simulink model "DCDCconverter"  (R2012b)
settings: Solver=ode3  StartTime=0.0  StopTime=inf  FixedStep=Tsample_simulink  RelTol=1e-3
PostLoadFcn:
  | , if any(exist('dsrtsu_mdlpostloadfcn', 'file') == [2, 3, 6]), try dsrtsu_mdlpostloadfcn('Execute', bdroot); catch fprintf('Error in PostLoadFcn (dsrtsu_mdlpostloadfcn) for model "%s":\n %s\n', bdroot, lasterr); end, end,
InitFcn:
  | load('../sim/me547_based_PI_controller_v3_saved_state.mat');
  | load('../sim/RuleBasedControlData_LiFe_76p8V_0C.mat');
undefined symbols (not defined in the file): BatVoltageLowerThresh, BatVoltageUpperThresh, C, DiscIntNeverNeededParam, Ea, fdesignblkfcn, gcbh, Icommand_Limit, Ireg_Integ_Limit, Kp_vc, MaxBatCurrent, MaxBatVoltage, MaxTemperature, MaxUCCurrent, MaxUCVoltage, Ra, RuleBasedControlHESSPowerValues, RuleBasedControlLUTValues, RuleBasedControlUCVoltageValues, TDelay_UltracapacitorRelay, Ts, Ts2, Tsample_simulink, UCVoltageLowerThresh, UCVoltageUpperThresh, Vbat, Vrail_rated
libraries: xpclib x35, rtilib1103 x8, dspsigops x5
(part 2 of 10)

== system DCDCconverter/RTI Data/RTI Data Store ==
  RTI Data Store : Subsystem  mask(RTI_DATA_STORE){}
      mask help:
      | RTI Data Store Block. This block is used by RTI to store internal model dependent data. Deleting this block will result in data loss.
      |
      | NEVER DELETE, COPY, OR MODIFY THIS BLOCK!
      mask Help:
      | RTI Data Store Block. This block is used by RTI to store internal model dependent data. Deleting this block will result in data loss.
      | 
      | NEVER DELETE, COPY, OR MODIFY THIS BLOCK!
      mask Display: text(0.5, 0.5, ' ', 'HorizontalAlignment', 'center');

== system DCDCconverter/Test Icmd/RuleBasedControlWithLUT ==
  HESSPower : Inport
  UCVoltage : Inport  Port=2
  2-D Lookup Table : Lookup_n-D  BreakpointsForDimension1=RuleBasedControlHESSPowerValues  BreakpointsForDimension2=RuleBasedControlUCVoltageValues  BreakpointsForDimension1Min=0  BreakpointsForDimension1Max=20000  Table=RuleBasedControlLUTValues  RndMeth=Simplest  InputSameDT=on
  MATLAB Function1 : MATLAB Function  TreatAsAtomicUnit=on
  Ra : Gain  Gain=-1
  Saturation : Saturate  UpperLimit=0  LowerLimit=-Icommand_Limit
  Switch2 : Switch  Threshold=1  OutDataTypeStr=Inherit: Inherit via back propagation
  UCCurrentCommand : Outport
  wires:
  HESSPower/1 -> MATLAB Function1/2(Pout), 2-D Lookup Table/1
  2-D Lookup Table/1 -> Ra/1
  MATLAB Function1/1(LUTEnabled) -> Switch2/2
  Switch2/1 -> UCCurrentCommand/1
  UCVoltage/1 -> MATLAB Function1/1(UCVoltage), 2-D Lookup Table/2
  MATLAB Function1/2(UCCurrentCommand) -> Switch2/3
  Ra/1 -> Saturation/1
  Saturation/1 -> Switch2/1

== system DCDCconverter/Circuit Outputs/Battery_Current/Lowpass Filter ==
  In : Inport
  Generated Filter Block : DiscreteFir  Tag=BlockMethodSubSystem  Coefficients=[0.00028387225120269494 -0.00039401751517345108 -0.00051440691195126409 -0.00075899521627574443 -0.0010941645666664886 -0.0015047026375922569 -0.0019783528421440672 -0.0024999962120832451 -0.0030483497757197702 -0.0035960077296140411 -0.0041083697578374141 -0.0045449722259694068 -0.0048595556741518183 -0.005002396212585635 -0.0049212033541306032 -0.0045644105295144241 -0.0038825540014864241 -0.0028320966661358709 -0.0013766635178792236 0.00050903213236998929 0.0028384532311130119 0.0056092612802153413 0.00880458302290015 0.012388421653013841 0.01631021984014288 0.020504166250900041 0.024885630758212381 0.029361560221717091 0.033828170940403357 0.03817500973917367 0.042289844667114912 0.046062416914275706 0.049388306387152664 0.052173366785398176 0.054337104315716686 0.055816180296302371 0.056566862063799822 0.056566862063799822 0.055816180296302371 0.054337104315716686 0.052173366785398176 0.049388306387152664 0.046062416914275706 0.042289844667114912 0.03817500973917367 0.033828170940403357 0.029361560221717091 0.024885630758212381 0.020504166250900041 0.01631021984014288 0.012388421653013841 0.00880458302290015 0.0056092612802153413 0.0028384532311130119 0.00050903213236998929 -0.0013766635178792236 -0.0028320966661358709 -0.0038825540014864241 -0.0045644105295144241 -0.0049212033541306032 -0.005002396212585635 -0.0048595556741518183 -0.0045449722259694068 -0.0041083697578374141 -0.0035960077296140411 -0.0030483497757197702 -0.0024999962120832451 -0.0019783528421440672 -0.0015047026375922569 -0.0010941645666664886 -0.00075899521627574443 -0.00051440691195126409 -0.00039401751517345108 0.00028387225120269494]  InputProcessing=Columns as channels (frame based)
  Out : Outport
  wires:
  In/1 -> Generated Filter Block/1
  Generated Filter Block/1 -> Out/1

== system DCDCconverter/Circuit Outputs/Battery_Voltage/Lowpass Filter ==
  In : Inport
  Generated Filter Block : DiscreteFir  Tag=BlockMethodSubSystem  Coefficients=[0.00028387225120269494 -0.00039401751517345108 -0.00051440691195126409 -0.00075899521627574443 -0.0010941645666664886 -0.0015047026375922569 -0.0019783528421440672 -0.0024999962120832451 -0.0030483497757197702 -0.0035960077296140411 -0.0041083697578374141 -0.0045449722259694068 -0.0048595556741518183 -0.005002396212585635 -0.0049212033541306032 -0.0045644105295144241 -0.0038825540014864241 -0.0028320966661358709 -0.0013766635178792236 0.00050903213236998929 0.0028384532311130119 0.0056092612802153413 0.00880458302290015 0.012388421653013841 0.01631021984014288 0.020504166250900041 0.024885630758212381 0.029361560221717091 0.033828170940403357 0.03817500973917367 0.042289844667114912 0.046062416914275706 0.049388306387152664 0.052173366785398176 0.054337104315716686 0.055816180296302371 0.056566862063799822 0.056566862063799822 0.055816180296302371 0.054337104315716686 0.052173366785398176 0.049388306387152664 0.046062416914275706 0.042289844667114912 0.03817500973917367 0.033828170940403357 0.029361560221717091 0.024885630758212381 0.020504166250900041 0.01631021984014288 0.012388421653013841 0.00880458302290015 0.0056092612802153413 0.0028384532311130119 0.00050903213236998929 -0.0013766635178792236 -0.0028320966661358709 -0.0038825540014864241 -0.0045644105295144241 -0.0049212033541306032 -0.005002396212585635 -0.0048595556741518183 -0.0045449722259694068 -0.0041083697578374141 -0.0035960077296140411 -0.0030483497757197702 -0.0024999962120832451 -0.0019783528421440672 -0.0015047026375922569 -0.0010941645666664886 -0.00075899521627574443 -0.00051440691195126409 -0.00039401751517345108 0.00028387225120269494]  InputProcessing=Columns as channels (frame based)
  Out : Outport
  wires:
  In/1 -> Generated Filter Block/1
  Generated Filter Block/1 -> Out/1

== system DCDCconverter/Circuit Outputs/Load_Current/Lowpass Filter ==
  In : Inport
  Generated Filter Block : DiscreteFir  Tag=BlockMethodSubSystem  Coefficients=[0.00028387225120269494 -0.00039401751517345108 -0.00051440691195126409 -0.00075899521627574443 -0.0010941645666664886 -0.0015047026375922569 -0.0019783528421440672 -0.0024999962120832451 -0.0030483497757197702 -0.0035960077296140411 -0.0041083697578374141 -0.0045449722259694068 -0.0048595556741518183 -0.005002396212585635 -0.0049212033541306032 -0.0045644105295144241 -0.0038825540014864241 -0.0028320966661358709 -0.0013766635178792236 0.00050903213236998929 0.0028384532311130119 0.0056092612802153413 0.00880458302290015 0.012388421653013841 0.01631021984014288 0.020504166250900041 0.024885630758212381 0.029361560221717091 0.033828170940403357 0.03817500973917367 0.042289844667114912 0.046062416914275706 0.049388306387152664 0.052173366785398176 0.054337104315716686 0.055816180296302371 0.056566862063799822 0.056566862063799822 0.055816180296302371 0.054337104315716686 0.052173366785398176 0.049388306387152664 0.046062416914275706 0.042289844667114912 0.03817500973917367 0.033828170940403357 0.029361560221717091 0.024885630758212381 0.020504166250900041 0.01631021984014288 0.012388421653013841 0.00880458302290015 0.0056092612802153413 0.0028384532311130119 0.00050903213236998929 -0.0013766635178792236 -0.0028320966661358709 -0.0038825540014864241 -0.0045644105295144241 -0.0049212033541306032 -0.005002396212585635 -0.0048595556741518183 -0.0045449722259694068 -0.0041083697578374141 -0.0035960077296140411 -0.0030483497757197702 -0.0024999962120832451 -0.0019783528421440672 -0.0015047026375922569 -0.0010941645666664886 -0.00075899521627574443 -0.00051440691195126409 -0.00039401751517345108 0.00028387225120269494]  InputProcessing=Columns as channels (frame based)
  Out : Outport
  wires:
  Generated Filter Block/1 -> Out/1
  In/1 -> Generated Filter Block/1

== system DCDCconverter/Circuit Outputs/UltraCapacitor_Current/Lowpass Filter ==
  In : Inport
  Generated Filter Block : DiscreteFir  Tag=BlockMethodSubSystem  Coefficients=[0.00028387225120269494 -0.00039401751517345108 -0.00051440691195126409 -0.00075899521627574443 -0.0010941645666664886 -0.0015047026375922569 -0.0019783528421440672 -0.0024999962120832451 -0.0030483497757197702 -0.0035960077296140411 -0.0041083697578374141 -0.0045449722259694068 -0.0048595556741518183 -0.005002396212585635 -0.0049212033541306032 -0.0045644105295144241 -0.0038825540014864241 -0.0028320966661358709 -0.0013766635178792236 0.00050903213236998929 0.0028384532311130119 0.0056092612802153413 0.00880458302290015 0.012388421653013841 0.01631021984014288 0.020504166250900041 0.024885630758212381 0.029361560221717091 0.033828170940403357 0.03817500973917367 0.042289844667114912 0.046062416914275706 0.049388306387152664 0.052173366785398176 0.054337104315716686 0.055816180296302371 0.056566862063799822 0.056566862063799822 0.055816180296302371 0.054337104315716686 0.052173366785398176 0.049388306387152664 0.046062416914275706 0.042289844667114912 0.03817500973917367 0.033828170940403357 0.029361560221717091 0.024885630758212381 0.020504166250900041 0.01631021984014288 0.012388421653013841 0.00880458302290015 0.0056092612802153413 0.0028384532311130119 0.00050903213236998929 -0.0013766635178792236 -0.0028320966661358709 -0.0038825540014864241 -0.0045644105295144241 -0.0049212033541306032 -0.005002396212585635 -0.0048595556741518183 -0.0045449722259694068 -0.0041083697578374141 -0.0035960077296140411 -0.0030483497757197702 -0.0024999962120832451 -0.0019783528421440672 -0.0015047026375922569 -0.0010941645666664886 -0.00075899521627574443 -0.00051440691195126409 -0.00039401751517345108 0.00028387225120269494]  InputProcessing=Columns as channels (frame based)
  Out : Outport
  wires:
  In/1 -> Generated Filter Block/1
  Generated Filter Block/1 -> Out/1

== system DCDCconverter/Circuit Outputs/UltraCapacitor_Voltage/Lowpass Filter ==
  In : Inport
  Generated Filter Block : DiscreteFir  Tag=BlockMethodSubSystem  Coefficients=[0.00028387225120269494 -0.00039401751517345108 -0.00051440691195126409 -0.00075899521627574443 -0.0010941645666664886 -0.0015047026375922569 -0.0019783528421440672 -0.0024999962120832451 -0.0030483497757197702 -0.0035960077296140411 -0.0041083697578374141 -0.0045449722259694068 -0.0048595556741518183 -0.005002396212585635 -0.0049212033541306032 -0.0045644105295144241 -0.0038825540014864241 -0.0028320966661358709 -0.0013766635178792236 0.00050903213236998929 0.0028384532311130119 0.0056092612802153413 0.00880458302290015 0.012388421653013841 0.01631021984014288 0.020504166250900041 0.024885630758212381 0.029361560221717091 0.033828170940403357 0.03817500973917367 0.042289844667114912 0.046062416914275706 0.049388306387152664 0.052173366785398176 0.054337104315716686 0.055816180296302371 0.056566862063799822 0.056566862063799822 0.055816180296302371 0.054337104315716686 0.052173366785398176 0.049388306387152664 0.046062416914275706 0.042289844667114912 0.03817500973917367 0.033828170940403357 0.029361560221717091 0.024885630758212381 0.020504166250900041 0.01631021984014288 0.012388421653013841 0.00880458302290015 0.0056092612802153413 0.0028384532311130119 0.00050903213236998929 -0.0013766635178792236 -0.0028320966661358709 -0.0038825540014864241 -0.0045644105295144241 -0.0049212033541306032 -0.005002396212585635 -0.0048595556741518183 -0.0045449722259694068 -0.0041083697578374141 -0.0035960077296140411 -0.0030483497757197702 -0.0024999962120832451 -0.0019783528421440672 -0.0015047026375922569 -0.0010941645666664886 -0.00075899521627574443 -0.00051440691195126409 -0.00039401751517345108 0.00028387225120269494]  InputProcessing=Columns as channels (frame based)
  Out : Outport
  wires:
  Generated Filter Block/1 -> Out/1
  In/1 -> Generated Filter Block/1

== system DCDCconverter/RTI Data/RTI Data Store/RTI Data Store ==
  RTI Data Store : Subsystem  mask(RTI_DATA_STORE){}
      mask help:
      | RTI Data Store Block. This block is used by RTI to store internal model dependent data. Deleting this block will result in data loss.
      |
      | NEVER DELETE, COPY, OR MODIFY THIS BLOCK!
      mask Help:
      | RTI Data Store Block. This block is used by RTI to store internal model dependent data. Deleting this block will result in data loss.
      | 
      | NEVER DELETE, COPY, OR MODIFY THIS BLOCK!
      mask Display: text(0.5, 0.5, ' ', 'HorizontalAlignment', 'center');

== system DCDCconverter/RTI Data/RTI Data Store/RTI Data Store/RTI Data Store ==
  RTI Data Store : Subsystem  mask(RTI_DATA_STORE){}
      mask help:
      | RTI Data Store Block. This block is used by RTI to store internal model dependent data. Deleting this block will result in data loss.
      |
      | NEVER DELETE, COPY, OR MODIFY THIS BLOCK!
      mask Help:
      | RTI Data Store Block. This block is used by RTI to store internal model dependent data. Deleting this block will result in data loss.
      | 
      | NEVER DELETE, COPY, OR MODIFY THIS BLOCK!
      mask Display: text(0.5, 0.5, ' ', 'HorizontalAlignment', 'center');

== system DCDCconverter/RTI Data/RTI Data Store/RTI Data Store/RTI Data Store/RTI Data Store ==

== matlab function DCDCconverter/Test Icmd/RuleBasedControlWithLUT/MATLAB Function1 ==
  data: LUTEnabled output; UCCurrentCommand output; UCVoltage input; Pout input
function [LUTEnabled, UCCurrentCommand] = fcn(UCVoltage, Pout)

if Pout>=0
    LUTEnabled = 1;
    UCCurrentCommand = 0;
    
else
    LUTEnabled = 0;
    
    PowerShareRatio = 0.8;
    PtoUC = -Pout*PowerShareRatio; % Ultracap must draw power, so polarity is reversed
    UCCurrentCommand = PtoUC/UCVoltage;
end

== matlab function DCDCconverter/ErrorLatchingFunction ==
  data: BatCurrentAlert input; LBatCurrentAlert output; UCCurrentAlert input; BatVoltageAlert input; UCVoltageAlert input; TempAlert input; ErrorHB1 input; ErrorHB2 input; ErrorHB3 input; OverTemp input; Error_Reset input; LUCCurrentAlert output; LBatVoltageAlert output; LUCVoltageAlert output; LTempAlert output; LErrorHB1 output; LErrorHB2 output; LErrorHB3 output; LOverTemp output
function [LBatCurrentAlert, LUCCurrentAlert, LBatVoltageAlert, LUCVoltageAlert, LTempAlert, LErrorHB1, LErrorHB2, LErrorHB3, LOverTemp] = fcn(BatCurrentAlert, UCCurrentAlert, BatVoltageAlert, UCVoltageAlert, TempAlert, ErrorHB1, ErrorHB2, ErrorHB3, OverTemp, Error_Reset)

persistent LLBatCurrentAlert LLUCCurrentAlert LLBatVoltageAlert LLUCVoltageAlert LLTempAlert LLErrorHB1 LLErrorHB2 LLErrorHB3 LLOverTemp;

if isempty(LLBatCurrentAlert)
    LLBatCurrentAlert = 0;
end
if isempty(LLUCCurrentAlert)
    LLUCCurrentAlert = 0;
end
if isempty(LLBatVoltageAlert)
    LLBatVoltageAlert = 0;
end
if isempty(LLUCVoltageAlert)
    LLUCVoltageAlert = 0;
end
if isempty(LLTempAlert)
    LLTempAlert = 0;
end
if isempty(LLErrorHB1)
    LLErrorHB1 = 0;
end
if isempty(LLErrorHB2)
    LLErrorHB2 = 0;
end
if isempty(LLErrorHB3)
    LLErrorHB3 = 0;
end
if isempty(LLOverTemp)
    LLOverTemp = 0;
end

if Error_Reset==0
    LLBatCurrentAlert = 0;
    LLUCCurrentAlert = 0;
    LLBatVoltageAlert = 0;
    LLUCVoltageAlert = 0;
    LLTempAlert = 0;
    LLErrorHB1 = 0;
    LLErrorHB2 = 0;
    LLErrorHB3 = 0;
    LLOverTemp = 0;
end

LLBatCurrentAlert = max(LLBatCurrentAlert, BatCurrentAlert);
LLUCCurrentAlert = max(LLUCCurrentAlert, UCCurrentAlert);
LLBatVoltageAlert = max(LLBatVoltageAlert, BatVoltageAlert);
LLUCVoltageAlert = max(LLUCVoltageAlert, UCVoltageAlert);
LLTempAlert = max(LLTempAlert, TempAlert);
LLErrorHB1 = max(LLErrorHB1, ErrorHB1);
LLErrorHB2 = max(LLErrorHB2, ErrorHB2);
LLErrorHB3 = max(LLErrorHB3, ErrorHB3);
LLOverTemp = max(LLOverTemp, OverTemp);

LBatCurrentAlert = LLBatCurrentAlert;
LUCCurrentAlert = LLUCCurrentAlert;
LBatVoltageAlert = LLBatVoltageAlert;
LUCVoltageAlert = LLUCVoltageAlert;
LTempAlert = LLTempAlert;
LErrorHB1 = LLErrorHB1;
LErrorHB2 = LLErrorHB2;
LErrorHB3 = LLErrorHB3;
LOverTemp = LLOverTemp;
